simulink model "forcecontrol_DOF3"  (R2024b)
settings: Solver=VariableStepAuto  StartTime=0.0  StopTime=0.6  RelTol=1e-3
undefined symbols (not defined in the file): X, Y, Z
libraries: sm_lib x40, nesl_utility x40
(part 2 of 2)

== system forcecontrol_DOF3/Lefet Robot/Left/Subsystem2 ==
  PS-Simulink Converter1 : nesl_utility/PS-Simulink Converter  PhysicalDomain=network_engine_domain  SubClassName=ps_output  LeftPortType=input  RightPortType=output  PseudoPeriodic=off  Frequencies=[]  VectorFormat=inherit  Unit=inherit  AffineConversion=off
  PS-Simulink Converter2 : nesl_utility/PS-Simulink Converter  PhysicalDomain=network_engine_domain  SubClassName=ps_output  LeftPortType=input  RightPortType=output  PseudoPeriodic=off  Frequencies=[]  VectorFormat=inherit  Unit=inherit  AffineConversion=off
  PS-Simulink Converter4 : nesl_utility/PS-Simulink Converter  PhysicalDomain=network_engine_domain  SubClassName=ps_output  LeftPortType=input  RightPortType=output  PseudoPeriodic=off  Frequencies=[]  VectorFormat=inherit  Unit=inherit  AffineConversion=off
  Point : sm_lib/Curves and Surfaces/Point  GraphicType=None  MarkerShape=Sphere  MarkerSize=10  GraphicVisPropType=SimpleVisualProperties  GraphicDiffuseColor=[0.5 0.5 0.5]  GraphicOpacity=1.0  GraphicSpecularColor=[0.5 0.5 0.5 1.0]  GraphicAmbientColor=[0.15 0.15 0.15 1.0]  GraphicEmissiveColor=[0.0 0.0 0.0 1.0]  GraphicShininess=75
  Product : Product
  Product1 : Product
  Spatial Contact Force : sm_lib/Forces and Torques/Spatial Contact Force  NormalForceType=SmoothSpringDamper  NormalStiffness=1e6  NormalStiffnessUnits=N/m  NormalDamping=1e3  NormalDampingUnits=N/(m/s)  NormalTransitionRegionWidth=1e-3  NormalTransitionRegionWidthUnits=m  FrictionType=SmoothStickSlip  CoefficientOfStaticFriction=0.5  CoefficientOfDynamicFriction=0.3  FrictionalCriticalVelocity=1e-3  FrictionalCriticalVelocityUnits=m/s  SenseContactSignal=on  SensePenetrationDepth=off  SenseSeparationDistance=off  SenseNormalForceMagnitude=on  SenseFrictionalForceMagnitude=on  SenseNormalVelocity=off  SenseTangentialVelocity=off  SenseContactBaseRotation=off  SenseContactBaseTranslation=off  SenseContactFollowerRotation=off  SenseContactFollowerTranslation=off  ZeroCrossDetectContactStartAndEnd=off
  Conn1 : PMIOPort  Side=Right
  Conn2 : PMIOPort  Port=2  Side=Left
  N : Outport
  Ff : Outport  Port=2
  wires:
  PS-Simulink Converter4/1 -> Product/2  "N"
  PS-Simulink Converter1/1 -> Product1/1, Product/1
  PS-Simulink Converter2/1 -> Product1/2  "Ff1"
  Product/1 -> N/1
  Product1/1 -> Ff/1
  connections:
  Spatial Contact Force/LConn1 -- Point/RConn1
  PS-Simulink Converter1/LConn1 -- Spatial Contact Force/RConn2
  PS-Simulink Converter4/LConn1 -- Spatial Contact Force/RConn3
  Conn1/RConn1 -- Spatial Contact Force/RConn1
  Point/LConn1 -- Conn2/RConn1
  PS-Simulink Converter2/LConn1 -- Spatial Contact Force/RConn4

== system forcecontrol_DOF3/Lefet Robot/Left/Subsystem3 ==
  PS-Simulink Converter1 : nesl_utility/PS-Simulink Converter  PhysicalDomain=network_engine_domain  SubClassName=ps_output  LeftPortType=input  RightPortType=output  PseudoPeriodic=off  Frequencies=[]  VectorFormat=inherit  Unit=inherit  AffineConversion=off
  PS-Simulink Converter2 : nesl_utility/PS-Simulink Converter  PhysicalDomain=network_engine_domain  SubClassName=ps_output  LeftPortType=input  RightPortType=output  PseudoPeriodic=off  Frequencies=[]  VectorFormat=inherit  Unit=inherit  AffineConversion=off
  PS-Simulink Converter4 : nesl_utility/PS-Simulink Converter  PhysicalDomain=network_engine_domain  SubClassName=ps_output  LeftPortType=input  RightPortType=output  PseudoPeriodic=off  Frequencies=[]  VectorFormat=inherit  Unit=inherit  AffineConversion=off
  Point : sm_lib/Curves and Surfaces/Point  GraphicType=None  MarkerShape=Sphere  MarkerSize=10  GraphicVisPropType=SimpleVisualProperties  GraphicDiffuseColor=[0.5 0.5 0.5]  GraphicOpacity=1.0  GraphicSpecularColor=[0.5 0.5 0.5 1.0]  GraphicAmbientColor=[0.15 0.15 0.15 1.0]  GraphicEmissiveColor=[0.0 0.0 0.0 1.0]  GraphicShininess=75
  Product : Product
  Product1 : Product
  Spatial Contact Force : sm_lib/Forces and Torques/Spatial Contact Force  NormalForceType=SmoothSpringDamper  NormalStiffness=1e6  NormalStiffnessUnits=N/m  NormalDamping=1e3  NormalDampingUnits=N/(m/s)  NormalTransitionRegionWidth=1e-3  NormalTransitionRegionWidthUnits=m  FrictionType=SmoothStickSlip  CoefficientOfStaticFriction=0.5  CoefficientOfDynamicFriction=0.3  FrictionalCriticalVelocity=1e-3  FrictionalCriticalVelocityUnits=m/s  SenseContactSignal=on  SensePenetrationDepth=off  SenseSeparationDistance=off  SenseNormalForceMagnitude=on  SenseFrictionalForceMagnitude=on  SenseNormalVelocity=off  SenseTangentialVelocity=off  SenseContactBaseRotation=off  SenseContactBaseTranslation=off  SenseContactFollowerRotation=off  SenseContactFollowerTranslation=off  ZeroCrossDetectContactStartAndEnd=off
  Conn1 : PMIOPort  Side=Right
  Conn2 : PMIOPort  Port=2  Side=Left
  N : Outport
  Ff : Outport  Port=2
  wires:
  PS-Simulink Converter4/1 -> Product/2  "N"
  PS-Simulink Converter1/1 -> Product1/1, Product/1
  PS-Simulink Converter2/1 -> Product1/2  "Ff1"
  Product/1 -> N/1
  Product1/1 -> Ff/1
  connections:
  Spatial Contact Force/LConn1 -- Point/RConn1
  PS-Simulink Converter1/LConn1 -- Spatial Contact Force/RConn2
  PS-Simulink Converter4/LConn1 -- Spatial Contact Force/RConn3
  Conn1/RConn1 -- Spatial Contact Force/RConn1
  Point/LConn1 -- Conn2/RConn1
  PS-Simulink Converter2/LConn1 -- Spatial Contact Force/RConn4

== system forcecontrol_DOF3/Lefet Robot/Left/Subsystem4 ==
  PS-Simulink Converter1 : nesl_utility/PS-Simulink Converter  PhysicalDomain=network_engine_domain  SubClassName=ps_output  LeftPortType=input  RightPortType=output  PseudoPeriodic=off  Frequencies=[]  VectorFormat=inherit  Unit=inherit  AffineConversion=off
  PS-Simulink Converter2 : nesl_utility/PS-Simulink Converter  PhysicalDomain=network_engine_domain  SubClassName=ps_output  LeftPortType=input  RightPortType=output  PseudoPeriodic=off  Frequencies=[]  VectorFormat=inherit  Unit=inherit  AffineConversion=off
  PS-Simulink Converter4 : nesl_utility/PS-Simulink Converter  PhysicalDomain=network_engine_domain  SubClassName=ps_output  LeftPortType=input  RightPortType=output  PseudoPeriodic=off  Frequencies=[]  VectorFormat=inherit  Unit=inherit  AffineConversion=off
  Point : sm_lib/Curves and Surfaces/Point  GraphicType=None  MarkerShape=Sphere  MarkerSize=10  GraphicVisPropType=SimpleVisualProperties  GraphicDiffuseColor=[0.5 0.5 0.5]  GraphicOpacity=1.0  GraphicSpecularColor=[0.5 0.5 0.5 1.0]  GraphicAmbientColor=[0.15 0.15 0.15 1.0]  GraphicEmissiveColor=[0.0 0.0 0.0 1.0]  GraphicShininess=75
  Product : Product
  Product1 : Product
  Spatial Contact Force : sm_lib/Forces and Torques/Spatial Contact Force  NormalForceType=SmoothSpringDamper  NormalStiffness=1e6  NormalStiffnessUnits=N/m  NormalDamping=1e3  NormalDampingUnits=N/(m/s)  NormalTransitionRegionWidth=1e-3  NormalTransitionRegionWidthUnits=m  FrictionType=SmoothStickSlip  CoefficientOfStaticFriction=0.5  CoefficientOfDynamicFriction=0.3  FrictionalCriticalVelocity=1e-3  FrictionalCriticalVelocityUnits=m/s  SenseContactSignal=on  SensePenetrationDepth=off  SenseSeparationDistance=off  SenseNormalForceMagnitude=on  SenseFrictionalForceMagnitude=on  SenseNormalVelocity=off  SenseTangentialVelocity=off  SenseContactBaseRotation=off  SenseContactBaseTranslation=off  SenseContactFollowerRotation=off  SenseContactFollowerTranslation=off  ZeroCrossDetectContactStartAndEnd=off
  Conn1 : PMIOPort  Side=Right
  Conn2 : PMIOPort  Port=2  Side=Left
  N : Outport
  Ff : Outport  Port=2
  wires:
  PS-Simulink Converter4/1 -> Product/2  "N"
  PS-Simulink Converter1/1 -> Product1/1, Product/1
  PS-Simulink Converter2/1 -> Product1/2  "Ff1"
  Product/1 -> N/1
  Product1/1 -> Ff/1
  connections:
  Spatial Contact Force/LConn1 -- Point/RConn1
  PS-Simulink Converter1/LConn1 -- Spatial Contact Force/RConn2
  PS-Simulink Converter4/LConn1 -- Spatial Contact Force/RConn3
  Conn1/RConn1 -- Spatial Contact Force/RConn1
  Point/LConn1 -- Conn2/RConn1
  PS-Simulink Converter2/LConn1 -- Spatial Contact Force/RConn4

== system forcecontrol_DOF3/Lefet Robot/Left/Subsystem5 ==
  PS-Simulink Converter1 : nesl_utility/PS-Simulink Converter  PhysicalDomain=network_engine_domain  SubClassName=ps_output  LeftPortType=input  RightPortType=output  PseudoPeriodic=off  Frequencies=[]  VectorFormat=inherit  Unit=inherit  AffineConversion=off
  PS-Simulink Converter2 : nesl_utility/PS-Simulink Converter  PhysicalDomain=network_engine_domain  SubClassName=ps_output  LeftPortType=input  RightPortType=output  PseudoPeriodic=off  Frequencies=[]  VectorFormat=inherit  Unit=inherit  AffineConversion=off
  PS-Simulink Converter4 : nesl_utility/PS-Simulink Converter  PhysicalDomain=network_engine_domain  SubClassName=ps_output  LeftPortType=input  RightPortType=output  PseudoPeriodic=off  Frequencies=[]  VectorFormat=inherit  Unit=inherit  AffineConversion=off
  Point : sm_lib/Curves and Surfaces/Point  GraphicType=None  MarkerShape=Sphere  MarkerSize=10  GraphicVisPropType=SimpleVisualProperties  GraphicDiffuseColor=[0.5 0.5 0.5]  GraphicOpacity=1.0  GraphicSpecularColor=[0.5 0.5 0.5 1.0]  GraphicAmbientColor=[0.15 0.15 0.15 1.0]  GraphicEmissiveColor=[0.0 0.0 0.0 1.0]  GraphicShininess=75
  Product : Product
  Product1 : Product
  Spatial Contact Force : sm_lib/Forces and Torques/Spatial Contact Force  NormalForceType=SmoothSpringDamper  NormalStiffness=1e6  NormalStiffnessUnits=N/m  NormalDamping=1e3  NormalDampingUnits=N/(m/s)  NormalTransitionRegionWidth=1e-3  NormalTransitionRegionWidthUnits=m  FrictionType=SmoothStickSlip  CoefficientOfStaticFriction=0.5  CoefficientOfDynamicFriction=0.3  FrictionalCriticalVelocity=1e-3  FrictionalCriticalVelocityUnits=m/s  SenseContactSignal=on  SensePenetrationDepth=off  SenseSeparationDistance=off  SenseNormalForceMagnitude=on  SenseFrictionalForceMagnitude=on  SenseNormalVelocity=off  SenseTangentialVelocity=off  SenseContactBaseRotation=off  SenseContactBaseTranslation=off  SenseContactFollowerRotation=off  SenseContactFollowerTranslation=off  ZeroCrossDetectContactStartAndEnd=off
  Conn1 : PMIOPort  Side=Right
  Conn2 : PMIOPort  Port=2  Side=Left
  N : Outport
  Ff : Outport  Port=2
  wires:
  PS-Simulink Converter4/1 -> Product/2  "N"
  PS-Simulink Converter1/1 -> Product1/1, Product/1
  PS-Simulink Converter2/1 -> Product1/2  "Ff1"
  Product/1 -> N/1
  Product1/1 -> Ff/1
  connections:
  Spatial Contact Force/LConn1 -- Point/RConn1
  PS-Simulink Converter1/LConn1 -- Spatial Contact Force/RConn2
  PS-Simulink Converter4/LConn1 -- Spatial Contact Force/RConn3
  Conn1/RConn1 -- Spatial Contact Force/RConn1
  Point/LConn1 -- Conn2/RConn1
  PS-Simulink Converter2/LConn1 -- Spatial Contact Force/RConn4

== system forcecontrol_DOF3/Lefet Robot/Left/Subsystem6 ==
  PS-Simulink Converter1 : nesl_utility/PS-Simulink Converter  PhysicalDomain=network_engine_domain  SubClassName=ps_output  LeftPortType=input  RightPortType=output  PseudoPeriodic=off  Frequencies=[]  VectorFormat=inherit  Unit=inherit  AffineConversion=off
  PS-Simulink Converter2 : nesl_utility/PS-Simulink Converter  PhysicalDomain=network_engine_domain  SubClassName=ps_output  LeftPortType=input  RightPortType=output  PseudoPeriodic=off  Frequencies=[]  VectorFormat=inherit  Unit=inherit  AffineConversion=off
  PS-Simulink Converter4 : nesl_utility/PS-Simulink Converter  PhysicalDomain=network_engine_domain  SubClassName=ps_output  LeftPortType=input  RightPortType=output  PseudoPeriodic=off  Frequencies=[]  VectorFormat=inherit  Unit=inherit  AffineConversion=off
  Point : sm_lib/Curves and Surfaces/Point  GraphicType=None  MarkerShape=Sphere  MarkerSize=10  GraphicVisPropType=SimpleVisualProperties  GraphicDiffuseColor=[0.5 0.5 0.5]  GraphicOpacity=1.0  GraphicSpecularColor=[0.5 0.5 0.5 1.0]  GraphicAmbientColor=[0.15 0.15 0.15 1.0]  GraphicEmissiveColor=[0.0 0.0 0.0 1.0]  GraphicShininess=75
  Product : Product
  Product1 : Product
  Spatial Contact Force : sm_lib/Forces and Torques/Spatial Contact Force  NormalForceType=SmoothSpringDamper  NormalStiffness=1e6  NormalStiffnessUnits=N/m  NormalDamping=1e3  NormalDampingUnits=N/(m/s)  NormalTransitionRegionWidth=1e-3  NormalTransitionRegionWidthUnits=m  FrictionType=SmoothStickSlip  CoefficientOfStaticFriction=0.5  CoefficientOfDynamicFriction=0.3  FrictionalCriticalVelocity=1e-3  FrictionalCriticalVelocityUnits=m/s  SenseContactSignal=on  SensePenetrationDepth=off  SenseSeparationDistance=off  SenseNormalForceMagnitude=on  SenseFrictionalForceMagnitude=on  SenseNormalVelocity=off  SenseTangentialVelocity=off  SenseContactBaseRotation=off  SenseContactBaseTranslation=off  SenseContactFollowerRotation=off  SenseContactFollowerTranslation=off  ZeroCrossDetectContactStartAndEnd=off
  Conn1 : PMIOPort  Side=Right
  Conn2 : PMIOPort  Port=2  Side=Left
  N : Outport
  Ff : Outport  Port=2
  wires:
  PS-Simulink Converter4/1 -> Product/2  "N"
  PS-Simulink Converter1/1 -> Product1/1, Product/1
  PS-Simulink Converter2/1 -> Product1/2  "Ff1"
  Product/1 -> N/1
  Product1/1 -> Ff/1
  connections:
  Spatial Contact Force/LConn1 -- Point/RConn1
  PS-Simulink Converter1/LConn1 -- Spatial Contact Force/RConn2
  PS-Simulink Converter4/LConn1 -- Spatial Contact Force/RConn3
  Conn1/RConn1 -- Spatial Contact Force/RConn1
  Point/LConn1 -- Conn2/RConn1
  PS-Simulink Converter2/LConn1 -- Spatial Contact Force/RConn4

== system forcecontrol_DOF3/Lefet Robot/Left/Subsystem7 ==
  PS-Simulink Converter1 : nesl_utility/PS-Simulink Converter  PhysicalDomain=network_engine_domain  SubClassName=ps_output  LeftPortType=input  RightPortType=output  PseudoPeriodic=off  Frequencies=[]  VectorFormat=inherit  Unit=inherit  AffineConversion=off
  PS-Simulink Converter2 : nesl_utility/PS-Simulink Converter  PhysicalDomain=network_engine_domain  SubClassName=ps_output  LeftPortType=input  RightPortType=output  PseudoPeriodic=off  Frequencies=[]  VectorFormat=inherit  Unit=inherit  AffineConversion=off
  PS-Simulink Converter4 : nesl_utility/PS-Simulink Converter  PhysicalDomain=network_engine_domain  SubClassName=ps_output  LeftPortType=input  RightPortType=output  PseudoPeriodic=off  Frequencies=[]  VectorFormat=inherit  Unit=inherit  AffineConversion=off
  Point : sm_lib/Curves and Surfaces/Point  GraphicType=None  MarkerShape=Sphere  MarkerSize=10  GraphicVisPropType=SimpleVisualProperties  GraphicDiffuseColor=[0.5 0.5 0.5]  GraphicOpacity=1.0  GraphicSpecularColor=[0.5 0.5 0.5 1.0]  GraphicAmbientColor=[0.15 0.15 0.15 1.0]  GraphicEmissiveColor=[0.0 0.0 0.0 1.0]  GraphicShininess=75
  Product : Product
  Product1 : Product
  Spatial Contact Force : sm_lib/Forces and Torques/Spatial Contact Force  NormalForceType=SmoothSpringDamper  NormalStiffness=1e6  NormalStiffnessUnits=N/m  NormalDamping=1e3  NormalDampingUnits=N/(m/s)  NormalTransitionRegionWidth=1e-3  NormalTransitionRegionWidthUnits=m  FrictionType=SmoothStickSlip  CoefficientOfStaticFriction=0.5  CoefficientOfDynamicFriction=0.3  FrictionalCriticalVelocity=1e-3  FrictionalCriticalVelocityUnits=m/s  SenseContactSignal=on  SensePenetrationDepth=off  SenseSeparationDistance=off  SenseNormalForceMagnitude=on  SenseFrictionalForceMagnitude=on  SenseNormalVelocity=off  SenseTangentialVelocity=off  SenseContactBaseRotation=off  SenseContactBaseTranslation=off  SenseContactFollowerRotation=off  SenseContactFollowerTranslation=off  ZeroCrossDetectContactStartAndEnd=off
  Conn1 : PMIOPort  Side=Right
  Conn2 : PMIOPort  Port=2  Side=Left
  N : Outport
  Ff : Outport  Port=2
  wires:
  PS-Simulink Converter4/1 -> Product/2  "N"
  PS-Simulink Converter1/1 -> Product1/1, Product/1
  PS-Simulink Converter2/1 -> Product1/2  "Ff1"
  Product/1 -> N/1
  Product1/1 -> Ff/1
  connections:
  Spatial Contact Force/LConn1 -- Point/RConn1
  PS-Simulink Converter1/LConn1 -- Spatial Contact Force/RConn2
  PS-Simulink Converter4/LConn1 -- Spatial Contact Force/RConn3
  Conn1/RConn1 -- Spatial Contact Force/RConn1
  Point/LConn1 -- Conn2/RConn1
  PS-Simulink Converter2/LConn1 -- Spatial Contact Force/RConn4

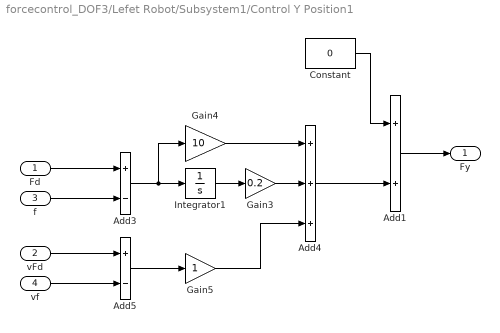
== system forcecontrol_DOF3/Lefet Robot/Subsystem1/Control Y Position1 ==
  Fd : Inport
  vFd : Inport  Port=2
  f : Inport  Port=3
  vf : Inport  Port=4
  Add1 : Sum
  Add3 : Sum  Inputs=+-
  Add4 : Sum  Inputs=+++
  Add5 : Sum  Inputs=+-
  Constant : Constant  Value=0
  Gain3 : Gain  Gain=0.2
  Gain4 : Gain  Gain=10
  Gain5 : Gain
  Integrator1 : Integrator
  Fy : Outport
  wires:
  vFd/1 -> Add5/1
  Add3/1 -> Gain4/1, Integrator1/1
  Gain3/1 -> Add4/2
  Fd/1 -> Add3/1
  vf/1 -> Add5/2
  Gain4/1 -> Add4/1
  Add5/1 -> Gain5/1
  Integrator1/1 -> Gain3/1
  Gain5/1 -> Add4/3
  f/1 -> Add3/2
  Add1/1 -> Fy/1
  Add4/1 -> Add1/2
  Constant/1 -> Add1/1

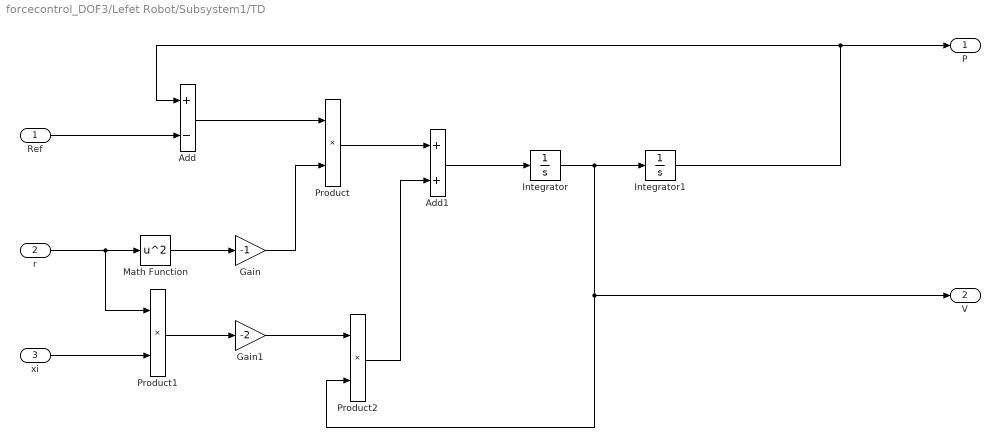
== system forcecontrol_DOF3/Lefet Robot/Subsystem1/TD ==
  Ref : Inport
  r : Inport  Port=2
  xi : Inport  Port=3
  Add : Sum  Inputs=+-
  Add1 : Sum
  Gain : Gain  Gain=-1
  Gain1 : Gain  Gain=-2
  Integrator : Integrator
  Integrator1 : Integrator
  Math Function : Math  Operator=square
  Product : Product
  Product1 : Product
  Product2 : Product
  P : Outport
  V : Outport  Port=2
  wires:
  Integrator/1 -> Product2/2, V/1, Integrator1/1
  Product1/1 -> Gain1/1
  Math Function/1 -> Gain/1
  Gain1/1 -> Product2/1
  Integrator1/1 -> Add/1, P/1
  Product2/1 -> Add1/2
  r/1 -> Product1/1, Math Function/1
  Product/1 -> Add1/1
  Add1/1 -> Integrator/1
  Add/1 -> Product/1
  Gain/1 -> Product/2
  xi/1 -> Product1/2
  Ref/1 -> Add/2

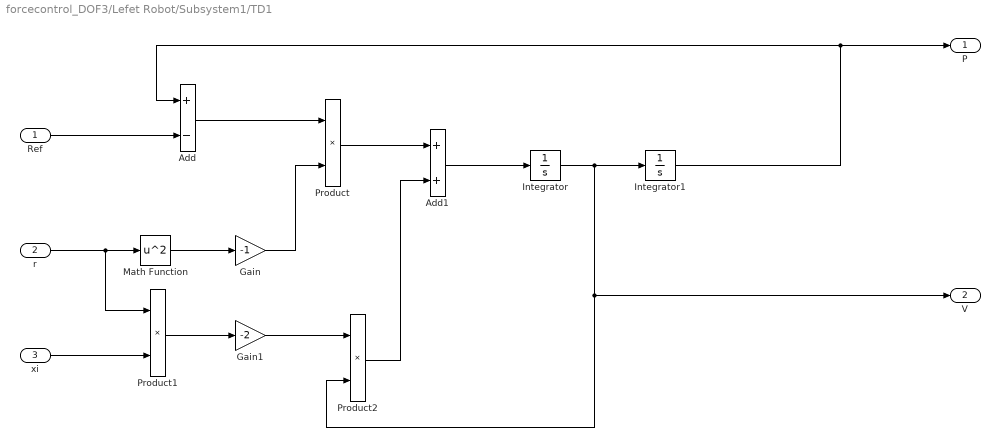
== system forcecontrol_DOF3/Lefet Robot/Subsystem1/TD1 ==
  Ref : Inport
  r : Inport  Port=2
  xi : Inport  Port=3
  Add : Sum  Inputs=+-
  Add1 : Sum
  Gain : Gain  Gain=-1
  Gain1 : Gain  Gain=-2
  Integrator : Integrator
  Integrator1 : Integrator
  Math Function : Math  Operator=square
  Product : Product
  Product1 : Product
  Product2 : Product
  P : Outport
  V : Outport  Port=2
  wires:
  Integrator/1 -> Product2/2, V/1, Integrator1/1
  Product1/1 -> Gain1/1
  Math Function/1 -> Gain/1
  Gain1/1 -> Product2/1
  Integrator1/1 -> Add/1, P/1
  Product2/1 -> Add1/2
  r/1 -> Product1/1, Math Function/1
  Product/1 -> Add1/1
  Add1/1 -> Integrator/1
  Add/1 -> Product/1
  Gain/1 -> Product/2
  xi/1 -> Product1/2
  Ref/1 -> Add/2

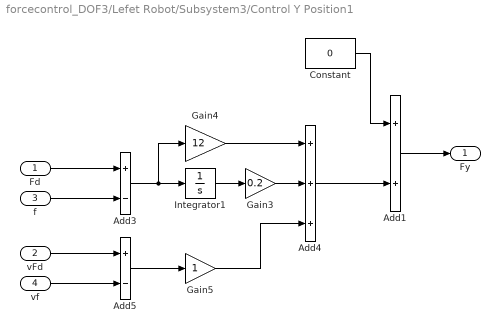
== system forcecontrol_DOF3/Lefet Robot/Subsystem3/Control Y Position1 ==
  Fd : Inport
  vFd : Inport  Port=2
  f : Inport  Port=3
  vf : Inport  Port=4
  Add1 : Sum
  Add3 : Sum  Inputs=+-
  Add4 : Sum  Inputs=+++
  Add5 : Sum  Inputs=+-
  Constant : Constant  Value=0
  Gain3 : Gain  Gain=0.2
  Gain4 : Gain  Gain=12
  Gain5 : Gain
  Integrator1 : Integrator
  Fy : Outport
  wires:
  vFd/1 -> Add5/1
  Add3/1 -> Gain4/1, Integrator1/1
  Gain3/1 -> Add4/2
  Fd/1 -> Add3/1
  vf/1 -> Add5/2
  Gain4/1 -> Add4/1
  Add5/1 -> Gain5/1
  Integrator1/1 -> Gain3/1
  Gain5/1 -> Add4/3
  f/1 -> Add3/2
  Add1/1 -> Fy/1
  Add4/1 -> Add1/2
  Constant/1 -> Add1/1

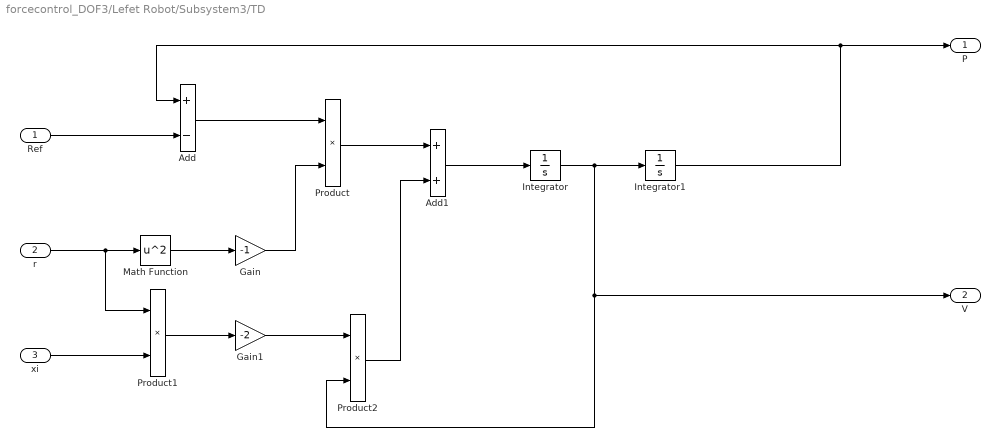
== system forcecontrol_DOF3/Lefet Robot/Subsystem3/TD ==
  Ref : Inport
  r : Inport  Port=2
  xi : Inport  Port=3
  Add : Sum  Inputs=+-
  Add1 : Sum
  Gain : Gain  Gain=-1
  Gain1 : Gain  Gain=-2
  Integrator : Integrator
  Integrator1 : Integrator
  Math Function : Math  Operator=square
  Product : Product
  Product1 : Product
  Product2 : Product
  P : Outport
  V : Outport  Port=2
  wires:
  Integrator/1 -> Product2/2, V/1, Integrator1/1
  Product1/1 -> Gain1/1
  Math Function/1 -> Gain/1
  Gain1/1 -> Product2/1
  Integrator1/1 -> Add/1, P/1
  Product2/1 -> Add1/2
  r/1 -> Product1/1, Math Function/1
  Product/1 -> Add1/1
  Add1/1 -> Integrator/1
  Add/1 -> Product/1
  Gain/1 -> Product/2
  xi/1 -> Product1/2
  Ref/1 -> Add/2

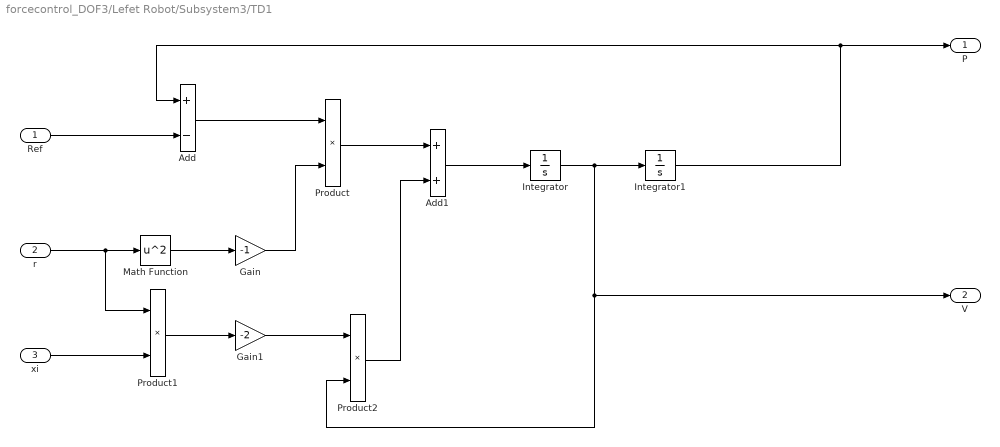
== system forcecontrol_DOF3/Lefet Robot/Subsystem3/TD1 ==
  Ref : Inport
  r : Inport  Port=2
  xi : Inport  Port=3
  Add : Sum  Inputs=+-
  Add1 : Sum
  Gain : Gain  Gain=-1
  Gain1 : Gain  Gain=-2
  Integrator : Integrator
  Integrator1 : Integrator
  Math Function : Math  Operator=square
  Product : Product
  Product1 : Product
  Product2 : Product
  P : Outport
  V : Outport  Port=2
  wires:
  Integrator/1 -> Product2/2, V/1, Integrator1/1
  Product1/1 -> Gain1/1
  Math Function/1 -> Gain/1
  Gain1/1 -> Product2/1
  Integrator1/1 -> Add/1, P/1
  Product2/1 -> Add1/2
  r/1 -> Product1/1, Math Function/1
  Product/1 -> Add1/1
  Add1/1 -> Integrator/1
  Add/1 -> Product/1
  Gain/1 -> Product/2
  xi/1 -> Product1/2
  Ref/1 -> Add/2

== system forcecontrol_DOF3/Lefet Robot/Subsystem4/Control Y Position1 ==
  Fd : Inport
  vFd : Inport  Port=2
  f : Inport  Port=3
  vf : Inport  Port=4
  Add1 : Sum
  Add3 : Sum  Inputs=+-
  Add4 : Sum  Inputs=+++
  Add5 : Sum  Inputs=+-
  Constant : Constant  Value=0
  Gain3 : Gain  Gain=0.2
  Gain4 : Gain  Gain=12
  Gain5 : Gain
  Integrator1 : Integrator
  Fy : Outport
  wires:
  vFd/1 -> Add5/1
  Add3/1 -> Gain4/1, Integrator1/1
  Gain3/1 -> Add4/2
  Fd/1 -> Add3/1
  vf/1 -> Add5/2
  Gain4/1 -> Add4/1
  Add5/1 -> Gain5/1
  Integrator1/1 -> Gain3/1
  Gain5/1 -> Add4/3
  f/1 -> Add3/2
  Add1/1 -> Fy/1
  Add4/1 -> Add1/2
  Constant/1 -> Add1/1

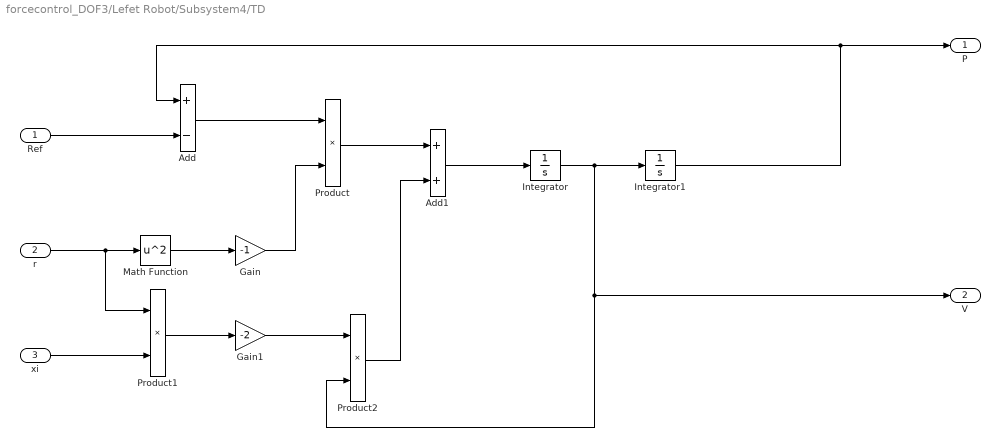
== system forcecontrol_DOF3/Lefet Robot/Subsystem4/TD ==
  Ref : Inport
  r : Inport  Port=2
  xi : Inport  Port=3
  Add : Sum  Inputs=+-
  Add1 : Sum
  Gain : Gain  Gain=-1
  Gain1 : Gain  Gain=-2
  Integrator : Integrator
  Integrator1 : Integrator
  Math Function : Math  Operator=square
  Product : Product
  Product1 : Product
  Product2 : Product
  P : Outport
  V : Outport  Port=2
  wires:
  Integrator/1 -> Product2/2, V/1, Integrator1/1
  Product1/1 -> Gain1/1
  Math Function/1 -> Gain/1
  Gain1/1 -> Product2/1
  Integrator1/1 -> Add/1, P/1
  Product2/1 -> Add1/2
  r/1 -> Product1/1, Math Function/1
  Product/1 -> Add1/1
  Add1/1 -> Integrator/1
  Add/1 -> Product/1
  Gain/1 -> Product/2
  xi/1 -> Product1/2
  Ref/1 -> Add/2

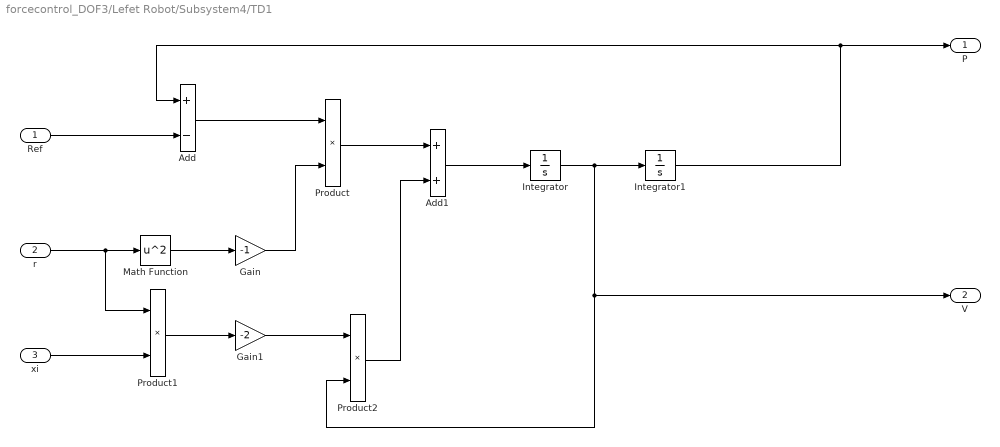
== system forcecontrol_DOF3/Lefet Robot/Subsystem4/TD1 ==
  Ref : Inport
  r : Inport  Port=2
  xi : Inport  Port=3
  Add : Sum  Inputs=+-
  Add1 : Sum
  Gain : Gain  Gain=-1
  Gain1 : Gain  Gain=-2
  Integrator : Integrator
  Integrator1 : Integrator
  Math Function : Math  Operator=square
  Product : Product
  Product1 : Product
  Product2 : Product
  P : Outport
  V : Outport  Port=2
  wires:
  Integrator/1 -> Product2/2, V/1, Integrator1/1
  Product1/1 -> Gain1/1
  Math Function/1 -> Gain/1
  Gain1/1 -> Product2/1
  Integrator1/1 -> Add/1, P/1
  Product2/1 -> Add1/2
  r/1 -> Product1/1, Math Function/1
  Product/1 -> Add1/1
  Add1/1 -> Integrator/1
  Add/1 -> Product/1
  Gain/1 -> Product/2
  xi/1 -> Product1/2
  Ref/1 -> Add/2

== matlab function forcecontrol_DOF3/Lefet Robot/MATLAB Function5 ==
  data: Ff1 input; Ff output; Ff2 input
function Ff = fcn(Ff1, Ff2)

Ff = mean(Ff1) + mean(Ff2);

== matlab function forcecontrol_DOF3/Lefet Robot/MATLAB Function ==
  data: u input; y output
function y = fcn(u)

if u<pi
    y = u;
else
    y = u - 2*pi;
end

== matlab function forcecontrol_DOF3/Lefet Robot/MATLAB Function2 ==
  data: tau1 output; q1 input; q2 input; q3 input; Fx input; Fy input; Fp input; tau2 output; tau3 output
function [tau1, tau2, tau3] = fcn(q1,q2,q3,Fx,Fy,Fp)
l1 = 0.5;
l2 = 0.5;
l3 = 0.1;

J = [-l1*sin(q1)-l2*sin(q1+q2)-l3*sin(q1+q2+q3),  -l2*sin(q1+q2)-l3*sin(q1+q2+q3),  -l3*sin(q1+q2+q3);
    l1*cos(q1)+l2*cos(q1+q2)+l3*cos(q1+q2+q3),  l2*cos(q1+q2)+l3*cos(q1+q2+q3),  l3*cos(q1+q2+q3);
    1,  1,  1];

% R = [cos(q1+q2+q3) -sin(q1+q2+q3) 0;
%     sin(q1+q2+q3) cos(q1+q2+q3) 0;
%     0 0 1];

tau = J'*[Fx; Fy; Fp];
tau1 = tau(1);
tau2 = tau(2);
tau3 = tau(3);

== matlab function forcecontrol_DOF3/Lefet Robot/MATLAB Function1 ==
  data: tau1 output; Q input
function tau1 = fcn(Q)

m1 = 0.125;
m2 = 0.125;
m3 = 0.009;
g = 9.80665;

l1 = 0.5/2;
l2 = 0.5/2;
l3 = 0.1/2;

q1 = Q(1);
q2 = Q(2);
q3 = Q(3);

tau1 = m3*g*(l1*cos(q1) + l2*cos(q1+q2) + l3*cos(q1+q2+q3)) + m2*g*(l1*cos(q1) + l2*cos(q1+q2)) + m1*g*l1*cos(q1);

== matlab function forcecontrol_DOF3/Lefet Robot/MATLAB Function3 ==
  data: tau2 output; Q input
function tau2 = fcn(Q)

m1 = 0.125;
m2 = 0.125;
m3 = 0.009;
g = 9.80665;

l1 = 0.5/2;
l2 = 0.5/2;
l3 = 0.1/2;

q1 = Q(1);
q2 = Q(2);
q3 = Q(3);

tau2 = m3*g*(l2*cos(q1+q2) + l3*cos(q1+q2+q3)) + m2*g*(l2*cos(q1+q2));

== matlab function forcecontrol_DOF3/Lefet Robot/MATLAB Function4 ==
  data: tau3 output; Q input
function tau3 = fcn(Q)

m1 = 0.125;
m2 = 0.125;
m3 = 0.009;
g = 9.80665;

l1 = 0.5/2;
l2 = 0.5/2;
l3 = 0.1/2;

q1 = Q(1);
q2 = Q(2);
q3 = Q(3);

tau3 = m3*g*(l3*cos(q1+q2+q3));

== matlab function forcecontrol_DOF3/Lefet Robot/MATLAB Function6 ==
  data: N1 input; Ff output; N2 input
function Ff = fcn(N1, N2)

Ff = mean(N1) + mean(N2);

== matlab function forcecontrol_DOF3/Lefet Robot/MATLAB Function8 ==
  data: N1 input; Tau output; N2 input
function Tau = fcn(N1, N2)


Tau = ((N1(1) + N1(3) + N2(1) + N2(3))/2 - (N1(2) + N1(4) + N2(2) + N2(4))/2)/0.04;
